simulink model "chatter"  (R2013a)
settings: Solver=ode45  StartTime=0.0  StopTime=100.0  RelTol=1e-3
undefined symbols (not defined in the file): k, m, mu, N, v, zv
libraries: simulink x1
settings Model: Creator=macuser  LastModifiedBy=macuser

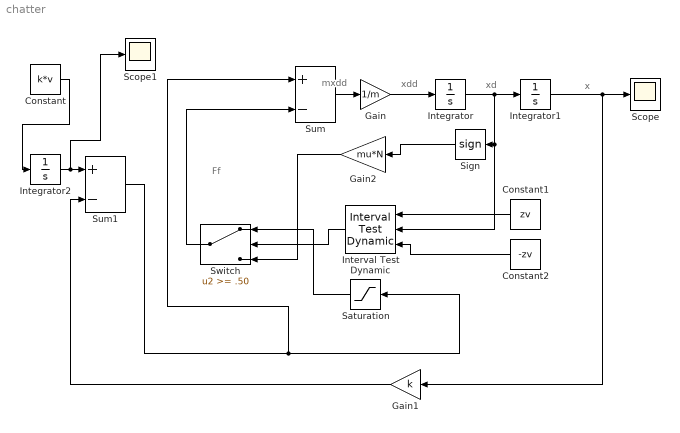
== system chatter ==
  note: Ff
  note: x
  note: xd
  note: xdd
  note: mxdd
  Constant : Constant  Value=k*v
  Constant1 : Constant  Value=zv
  Constant2 : Constant  Value=-zv
  Gain : Gain  Gain=1/m
  Gain1 : Gain  Gain=k
  Gain2 : Gain  Gain=mu*N
  Integrator : Integrator
  Integrator1 : Integrator
  Integrator2 : Integrator
  Interval Test Dynamic : simulink/Logic and Bit Operations/Interval Test Dynamic  IntervalClosedRight=on  IntervalClosedLeft=on  OutDataTypeStr=uint8
  Saturation : Saturate  UpperLimit=mu*N  LowerLimit=-mu*N
  Scope : Scope
  Scope1 : Scope
  Sign : Signum
  Sum : Sum  Inputs=+-
  Sum1 : Sum  Inputs=+-
  Switch : Switch  Threshold=.50
  wires:
  Sum/1 -> Gain/1
  Gain/1 -> Integrator/1
  Integrator/1 -> Interval Test Dynamic/2, Sign/1, Integrator1/1
  Integrator1/1 -> Gain1/1, Scope/1
  Constant/1 -> Integrator2/1
  Integrator2/1 -> Scope1/1, Sum1/1
  Gain1/1 -> Sum1/2
  Sum1/1 -> Sum/1, Saturation/1
  Sign/1 -> Gain2/1
  Constant1/1 -> Interval Test Dynamic/1
  Constant2/1 -> Interval Test Dynamic/3
  Interval Test Dynamic/1 -> Switch/2
  Saturation/1 -> Switch/1
  Gain2/1 -> Switch/3
  Switch/1 -> Sum/2
